simulink model "Project7"  (R2014a)
settings: Solver=ode3  StartTime=0.0  StopTime=Sim_Time  FixedStep=0.01  RelTol=1e-3
values from neighbouring files (symbols this model uses):
  b = 10    [Project7_Run.m]
  k = 20    [Project7_Run.m]
  Kd = 50    [Project7_Run.m]
  Ki = 300    [Project7_Run.m]
  Kp = 350    [Project7_Run.m]
  M = 1    [Project7_Run.m]
  Step_Value = 1    [Project7_Run.m]
settings Model: Creator=DZR3QN  LastModifiedBy=DZR3QN

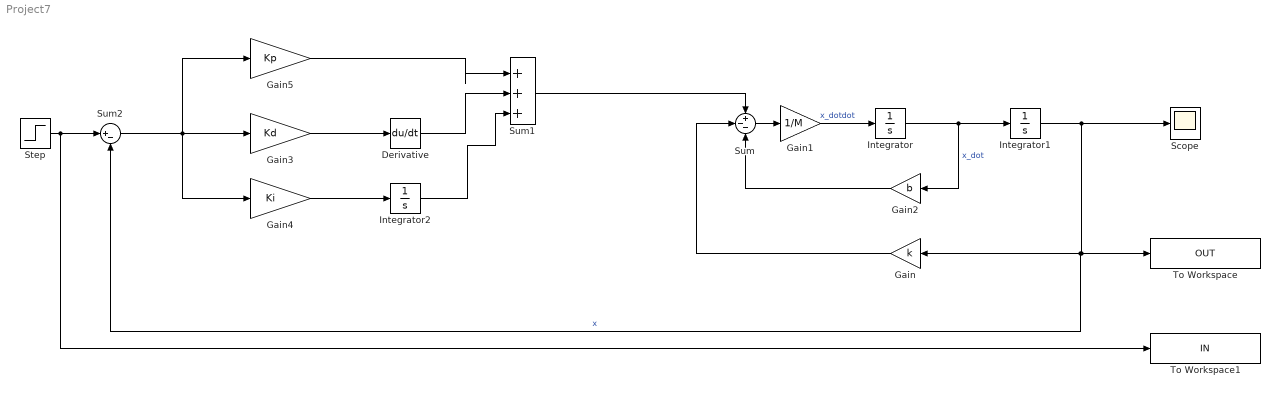
== system Project7 ==
  Derivative : Derivative
  Gain : Gain  Gain=k
  Gain1 : Gain  Gain=1/M
  Gain2 : Gain  Gain=b
  Gain3 : Gain  Gain=Kd
  Gain4 : Gain  Gain=Ki
  Gain5 : Gain  Gain=Kp
  Integrator : Integrator
  Integrator1 : Integrator
  Integrator2 : Integrator
  Scope : Scope
      settings: MaxDataPoints=50000
  Step : Step  After=Step_Value  SampleTime=0
  Sum : Sum  Inputs=+--
  Sum1 : Sum  Inputs=|+++
  Sum2 : Sum  Inputs=|+-
  To Workspace : ToWorkspace  VariableName=OUT  SaveFormat=Timeseries  SampleTime=-1
  To Workspace1 : ToWorkspace  VariableName=IN  SaveFormat=Timeseries  SampleTime=-1
  wires:
  Integrator/1 -> Gain2/1, Integrator1/1  "x_dot"
  Integrator1/1 -> Scope/1, Sum2/2, Gain/1, To Workspace/1  "x"
  Sum/1 -> Gain1/1
  Gain1/1 -> Integrator/1  "x_dotdot"
  Gain2/1 -> Sum/3
  Gain/1 -> Sum/2
  Sum1/1 -> Sum/1
  Derivative/1 -> Sum1/2
  Gain5/1 -> Sum1/1
  Sum2/1 -> Gain4/1, Gain5/1, Gain3/1
  Gain3/1 -> Derivative/1
  Gain4/1 -> Integrator2/1
  Integrator2/1 -> Sum1/3
  Step/1 -> To Workspace1/1, Sum2/1
